simulink model "realtime_test"  (R2025b)
settings: Solver=ode1be  StartTime=0.0  StopTime=1264/3840  FixedStep=1/3840  RelTol=1e-3
libraries: deeplib x1
settings Model: Creator=faizshaikh  LastModifiedBy=faizshaikh

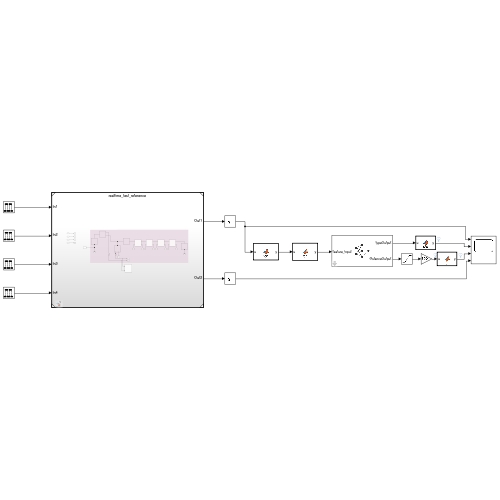
[thumbnail: Simulink's stored preview of the top-level diagram]
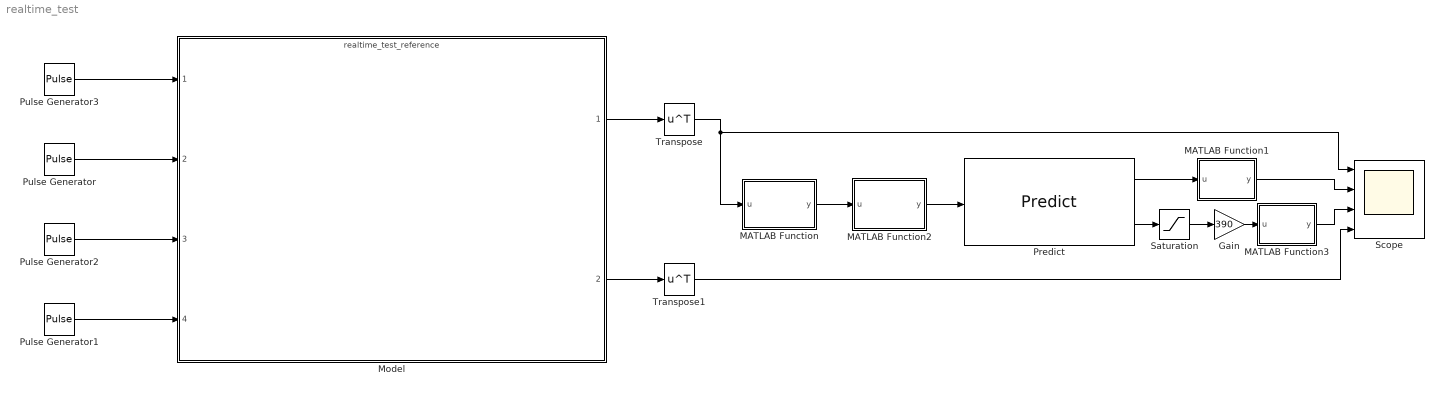
== system realtime_test ==
  Gain : Gain  Gain=390
  MATLAB Function : MATLAB Function  TreatAsAtomicUnit=on
  MATLAB Function1 : MATLAB Function  TreatAsAtomicUnit=on
  MATLAB Function2 : MATLAB Function  TreatAsAtomicUnit=on
  MATLAB Function3 : MATLAB Function  TreatAsAtomicUnit=on
  Model : ModelReference  ModelNameDialog=realtime_test_reference.slx  SimulationMode=Normal  ModelReferenceVersion=1.7
  Predict : deeplib/Predict  Network=Network from MAT-file  NetworkFunction=squeezenet  NetworkFilePath=/Users/faizshaikh/Documents/MATLAB/transmission_system/my_model_new.mat  MiniBatchSize=128  InputDataFormats={'feature_input', 'SSC';}  Predictions=on  Activations={}  ForceInterpretedSim=off  EnableDLNetwork=on  LastKnownNetworkFilePath='/Users/faizshaikh/Documents/MATLAB/transmission_system/my_model_new.mat'  LastKnownNetworkTimeStamp=740069.544699074118398129940032958984375
  Pulse Generator : DiscretePulseGenerator  Period=2468  PulseWidth=241  PhaseDelay=361  SampleTime=1/3840
  Pulse Generator1 : DiscretePulseGenerator  Period=2468  PulseWidth=241  PhaseDelay=963  SampleTime=1/3840
  Pulse Generator2 : DiscretePulseGenerator  Period=2468  PulseWidth=241  PhaseDelay=662  SampleTime=1/3840
  Pulse Generator3 : DiscretePulseGenerator  Period=2468  PulseWidth=241  PhaseDelay=60  SampleTime=1/3840
  Saturation : Saturate  UpperLimit=400  LowerLimit=0
  Scope : Scope  NumInputPorts=4
      settings: ActiveDisplayYMinimum=-0.49999999999999989  ActiveDisplayYMaximum=4.5
  Transpose : Math  Operator=transpose
  Transpose1 : Math  Operator=transpose
  wires:
  Model/1 -> Transpose/1
  Model/2 -> Transpose1/1
  Transpose/1 -> Scope/1, MATLAB Function/1(u)
  Transpose1/1 -> Scope/4
  Predict/1 -> MATLAB Function1/1(u)
  MATLAB Function1/1(y) -> Scope/2
  MATLAB Function2/1(y) -> Predict/1
  MATLAB Function/1(y) -> MATLAB Function2/1(u)
  Predict/2 -> Saturation/1
  Saturation/1 -> Gain/1
  Gain/1 -> MATLAB Function3/1(u)
  Pulse Generator/1 -> Model/2
  Pulse Generator3/1 -> Model/1
  Pulse Generator2/1 -> Model/3
  Pulse Generator1/1 -> Model/4
  MATLAB Function3/1(y) -> Scope/3

== matlab function realtime_test/MATLAB Function ==
  settings: updateMethod=DISCRETE
  data: u input; y output
function y = fcn(u)
    % persistent variables stay in memory between function calls
    persistent dataWindow count;
    
    % 1. Initialization
    if isempty(dataWindow)
        dataWindow = zeros(length(u), 301); 
        count = 0;
    end
    
    % 2. Increment counter and place the new sample in the next available slot
    count = count + 1;
    dataWindow(:, count) = u;
    
    % 3. Check if we have a full "page" of 321 samples
    if count >= 301
        y = dataWindow;
        dataWindow = zeros(size(dataWindow));
        count = 0;       
    else
        y = zeros(size(dataWindow)); 
    end
end

== matlab function realtime_test/MATLAB Function1 ==
  settings: updateMethod=DISCRETE
  data: u input; y output
function y = fcn(u)
    persistent offset_count;

    if isempty(offset_count)
        offset_count = 0;
    end

    if offset_count >= 300
        [~, winnerIdx] = max(u);
        if winnerIdx == 5
            y = 0; % Specific logic for index 5
        else
            y = winnerIdx;
        end
        offset_count = 0;
    else
        y = 0;
        offset_count = offset_count + 1;
    end
end

== matlab function realtime_test/MATLAB Function2 ==
  data: u input; y output
function y = fcn(u)
    a = u(1,:);
    b = u(2,:);
    c = u(3,:);
    Ig = a + b + c;
    d1 = modwt(a, 'db4');
    d2 = modwt(b, 'db4');
    d3 = modwt(c, 'db4');
    f = [Ig; d1(1,:); d2(1,:); d3(1,:)];
    y = sign(f) .* log10(abs(f) + 1e-15);
end

== matlab function realtime_test/MATLAB Function3 ==
  settings: updateMethod=DISCRETE
  data: u input; y output
function y = fcn(u)
    persistent offset_count;

    if isempty(offset_count)
        offset_count = 0;
    end

    if offset_count >= 300
        y = u;
        offset_count = 0;
    else
        y = u - 1.3625471e+02;
        offset_count = offset_count + 1;
    end
end
